simulink model "SimulinkValveControlv1"  (R2020b)
settings: Solver=VariableStepAuto  StartTime=0.0  StopTime=10.0  RelTol=1e-3
libraries: simulink x1
settings Model: Creator=ethan  LastModifiedBy=ethan

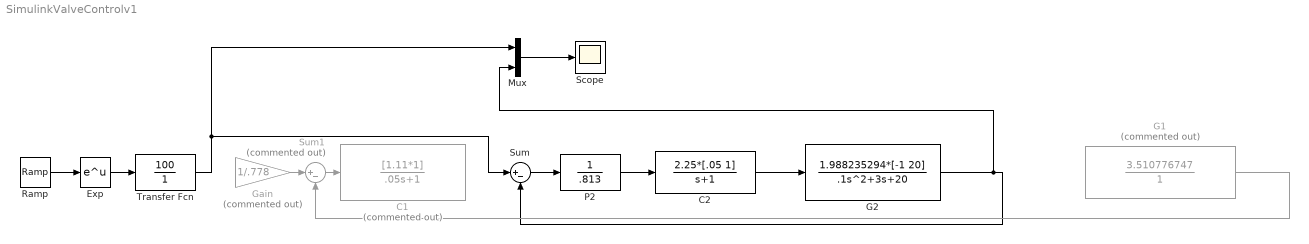
== system SimulinkValveControlv1 ==
  C1 : TransferFcn  Commented=on  Numerator=[1.11*1]  Denominator=[.05 1]
  C2 : TransferFcn  Numerator=2.25*[.05 1]  Denominator=[1 1]
  Exp : Math  SaturateOnIntegerOverflow=on
  G1 : TransferFcn  Commented=on  Numerator=[3.510776747]  Denominator=[1]
  G2 : TransferFcn  Numerator=1.988235294*[-1 20]  Denominator=[.1 3 20]
  Gain : Gain  Commented=on  Gain=1/.778
  Mux : Mux  Inputs=2
  P2 : TransferFcn  Denominator=[.813]
  Ramp : simulink/Sources/Ramp  slope=-.2  start=0  InitialOutput=0
  Scope : Scope
  Sum : Sum  Inputs=|+-
  Sum1 : Sum  Commented=on  Inputs=|+-
  Transfer Fcn : TransferFcn  Numerator=[100]  Denominator=[1]
  wires:
  C2/1 -> G2/1
  G2/1 -> Mux/2, Sum/2
  G1/1 -> Sum1/2
  Sum/1 -> P2/1
  P2/1 -> C2/1
  Ramp/1 -> Exp/1
  Exp/1 -> Transfer Fcn/1
  Transfer Fcn/1 -> Sum/1, Mux/1
  Mux/1 -> Scope/1
  Sum1/1 -> C1/1
  Gain/1 -> Sum1/1
